simulink model "WiFi"  (Simulink 5.0)
settings: Solver=VariableStepDiscrete  StartTime=0.0  StopTime=inf  RelTol=1e-3
PreLoadFcn:
  | EsNo=18; Distance=.1;
undefined symbols (not defined in the file): CRC_size, Filter_order, Fs, Length_size, Packet_size, PLCP_header_receive_delay, PLCP_header_size, PLCP_preamble_receive_delay, PLCP_preamble_size, PLCP_size, PPDU_frame_period, PPDU_size_chips, PSDU_receive_delay, PSDU_size, randint, Samples_per_chips, Service_size, SFD_size, Signal_size, Sync_bits, Sync_size
libraries: WiFi_lib x8, dspsrcs4 x6, commsink2 x5, dspsigops x4, simulink x3, dspsnks4 x1, dsparch3 x1, commutil2 x1, commrandsrc2 x1, dspmlti3 x1, dspstat3 x1
settings Model: Creator=Stuart Amit  LastModifiedBy=stuartm  SaveTime=off  SaveOutput=off  BooleanDataType=off

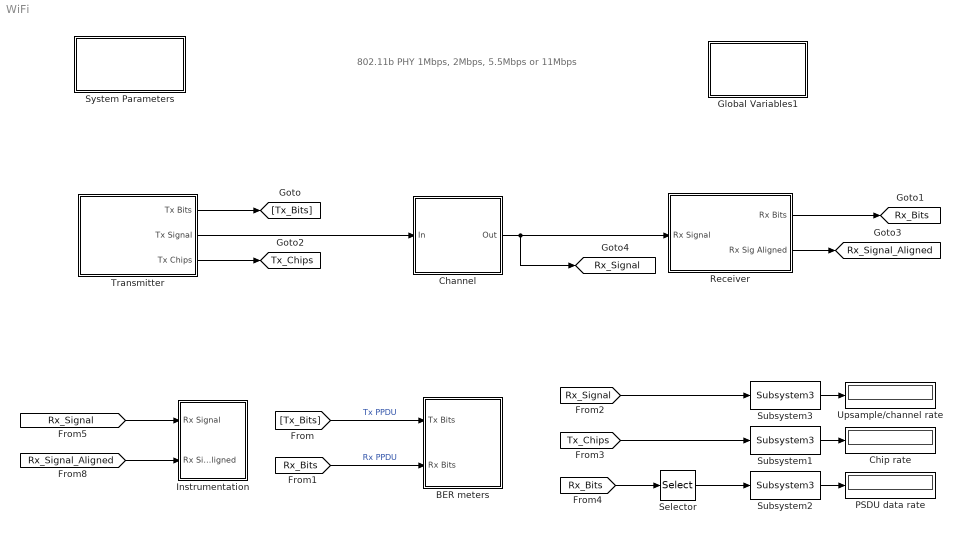
== system WiFi ==
  note: 802.11b PHY
      |   1Mbps, 2Mbps, 5.5Mbps or 11Mbps
  BER meters : Subsystem
  Channel : Subsystem  BlockChoice=AWGN
      settings: AttributesFormatString=%<BlockChoice>  TemplateBlock=WiFi_lib/Channel  MemberBlocks=AWGN,None
  Chip rate : Display
  Global Variables1 : Subsystem
      mask Display: disp('Info')
  Instrumentation : Subsystem  TreatAsAtomicUnit=on  mask(Instrumentation){On=off, Off=on}
      mask init:
      | if strcmp(On,'on')
      |   picture=imread('Switch_On.jpg');
      |   set_param([gcb,'/State'],'Value','1');
      | else
      |   picture=imread('Switch_Off.jpg');
      |   set_param([gcb,'/State'],'Value','0');
      | end
      settings: OpenFcn=temp=get_param(gcb,'On');set_param(gcb,'On', get_param(gcb,'Off'));set_param(gcb,'Off', temp);
      mask Display: image(picture,'center')
  PSDU data rate : Display
  Receiver : Subsystem
  Selector : Selector  Elements=[1: PSDU_size]  InputPortWidth=PPDU_size
  Subsystem1 : WiFi_lib/Subsystem3  Units=MHz
  Subsystem2 : WiFi_lib/Subsystem3  Units=MHz
  Subsystem3 : WiFi_lib/Subsystem3  Units=MHz
  System Parameters : Subsystem  mask(Set System Parameters){Mode=11Mbps, Packet_size=1024, Short_preamble=off, Channel_number=11, Channel_type=AWGN, EsNo=EsNo}
      mask prompts: Mode "Mode/Data Rate"; Packet_size "Packet Size (Bytes)"; Short_preamble "Use Short Preamble"; Channel_number "Channel Number"; Channel_type "Channel Type"; EsNo "Channel EsNo"
      mask help: These system parameters set-up configurable subsystems in the model to implmentedort the requested parameters. Calls wifi_init.m to perfom this task as well as calculate delays.
      mask init:
      | WiFi_init
      settings: AttributesFormatString="Rate = %<Mode>\\nPacket Size = %<Packet_size> Bytes\\nShort Preamble is %<Short_preamble>\\nChannel Number = %<Channel_number>\\nChannel Type =  %<Channel_type>\\nChannel Noise (EsNo) =  %<EsNo> dB\\n"
      mask StyleString: popup(1Mbps|2Mbps|5.5Mbps|11Mbps),edit,checkbox,popup(1|2|3|4|5|6|7|8|9|10|11),popup(None|AWGN),edit
      mask CallbackString:
      | ||||if strcmp(get_param(gcb,'Channel_type'),'AWGN')
      | 	set_param(gcb,'MaskEnables',{'on' 'on' 'on' 'on' 'on' 'on'})
      | else
      | 	set_param(gcb,'MaskEnables',{'on' 'on' 'on' 'on' 'on' 'off'})
      | end
      | 	|
      mask Display: disp('System Parameters')
  Transmitter : Subsystem
  Upsample/channel rate : Display
  tag scope: Rx_Bits=global, Rx_Signal=global, Rx_Signal_Aligned=global, Tx_Chips=global
  wires:
  Transmitter/2(Tx Signal) -> Channel/1(In)
  Transmitter/1(Tx Bits) -> [Tx_Bits]
  Receiver/1(Rx Bits) -> [Rx_Bits]
  [Rx_Bits] -> BER meters/2(Rx Bits)  "Rx PPDU"
  [Tx_Bits] -> BER meters/1(Tx Bits)  "Tx PPDU"
  Channel/1(Out) -> Receiver/1(Rx Signal), [Rx_Signal]
  Subsystem3/1 -> Upsample/channel rate/1
  [Rx_Signal] -> Subsystem3/1
  Subsystem1/1 -> Chip rate/1
  [Tx_Chips] -> Subsystem1/1
  [Rx_Bits] -> Selector/1
  Subsystem2/1 -> PSDU data rate/1
  Selector/1 -> Subsystem2/1
  Receiver/2(Rx Sig Aligned) -> [Rx_Signal_Aligned]
  [Rx_Signal_Aligned] -> Instrumentation/2(Rx Signal Aligned)
  [Rx_Signal] -> Instrumentation/1(Rx Signal)
  Transmitter/3(Tx Chips) -> [Tx_Chips]

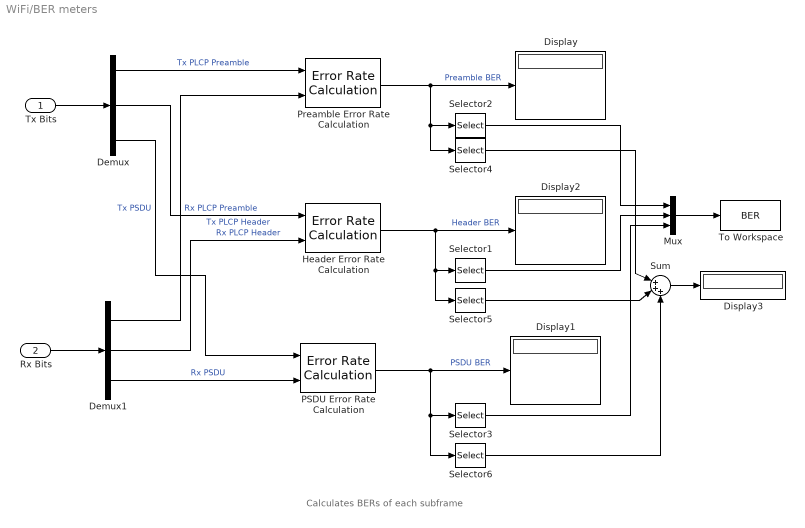
== system WiFi/BER meters ==
  note: Calculates BERs of each subframe
  Tx Bits : Inport
  Rx Bits : Inport  Port=2
  Demux : Demux  Outputs=[PLCP_preamble_size PLCP_header_size PSDU_size]
  Demux1 : Demux  Outputs=[PLCP_preamble_size PLCP_header_size PSDU_size]
  Display{,1..3} (4 alike) : Display
  Header Error Rate Calculation : commsink2/Error Rate Calculation  N=PLCP_header_receive_delay  st_delay=PLCP_header_computation_delay  cp_mode=Entire frame  subframe=3:4808  PMode=Port  WsName=ErrorVec  RsMode2=off  stop=off  numErr=100  maxBits=1e6
  Mux : Mux  Inputs=3
  PSDU Error Rate Calculation : commsink2/Error Rate Calculation  N=PSDU_receive_delay  st_delay=PSDU_computation_delay  cp_mode=Entire frame  subframe=3:4808  PMode=Port  WsName=ErrorVec  RsMode2=off  stop=on  numErr=100  maxBits=1e6
  Preamble Error Rate Calculation : commsink2/Error Rate Calculation  N=PLCP_preamble_receive_delay  st_delay=PLCP_preamble_computation_delay  cp_mode=Entire frame  subframe=3:4808  PMode=Port  WsName=ErrorVec  RsMode2=off  stop=off  numErr=100  maxBits=1e6
  Selector1 : Selector  Elements=[1]  InputPortWidth=3
  Selector2 : Selector  Elements=[1]  InputPortWidth=3
  Selector3 : Selector  Elements=[1]  InputPortWidth=3
  Selector4 : Selector  Elements=3  InputPortWidth=3
  Selector5 : Selector  Elements=3  InputPortWidth=3
  Selector6 : Selector  Elements=3  InputPortWidth=3
  Sum : Sum  Inputs=|+++  SaturateOnIntegerOverflow=on  InputSameDT=on
  To Workspace : ToWorkspace  VariableName=BER  SampleTime=-1  SaveFormat=Array
      settings: MaxDataPoints=1
  wires:
  Preamble Error Rate Calculation/1 -> Display/1, Selector2/1, Selector4/1  "Preamble BER"
  PSDU Error Rate Calculation/1 -> Display1/1, Selector3/1, Selector6/1  "PSDU BER"
  Demux1/1 -> Preamble Error Rate Calculation/2  "Rx PLCP Preamble"
  Demux/1 -> Preamble Error Rate Calculation/1  "Tx PLCP Preamble"
  Header Error Rate Calculation/1 -> Display2/1, Selector1/1, Selector5/1  "Header BER"
  Demux1/3 -> PSDU Error Rate Calculation/2  "Rx PSDU"
  Demux/3 -> PSDU Error Rate Calculation/1  "Tx PSDU"
  Demux/2 -> Header Error Rate Calculation/1  "Tx PLCP Header"
  Demux1/2 -> Header Error Rate Calculation/2  "Rx PLCP Header"
  Tx Bits/1 -> Demux/1
  Rx Bits/1 -> Demux1/1
  Selector2/1 -> Mux/1
  Mux/1 -> To Workspace/1
  Selector1/1 -> Mux/2
  Selector3/1 -> Mux/3
  Sum/1 -> Display3/1
  Selector4/1 -> Sum/1
  Selector5/1 -> Sum/2
  Selector6/1 -> Sum/3

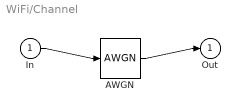
== system WiFi/Channel ==
  In : Inport
  AWGN : WiFi_lib/AWGN
  Out : Outport
  wires:
  In/1 -> AWGN/1
  AWGN/1 -> Out/1

== system WiFi/Global Variables1 ==
  note: Implements: IEEE Std 802.11b-1999 PHY
      | (Supplement to ANSI/IEEE Std 802.11, 1999 Edition)
      | Available from: http://standards.ieee.org/reading/ieee/std/lanman/
      |
      | System Parameters: Double click block to display and set
      |
      | * Mode/Data Rate: Choose from 1Mpbs, 2Mbps, 5.5Mbps or 11Mbps
      | * Packet size: 1-4095 Bytes
      | * Use short preamble: An option for 2, 5.5 or 11Mbps options only
      | * Channel number: Select from 1 to 11
      | * Channel type: None or AWGN
      | * EsNo: Channel noise power for AWGN option

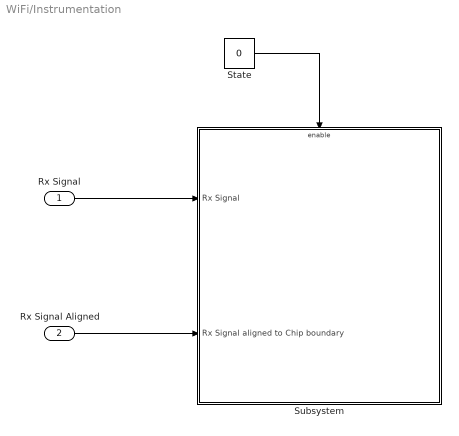
== system WiFi/Instrumentation ==
  Rx Signal : Inport
  Rx Signal Aligned : Inport  Port=2
  State : Constant  Value=0
  Subsystem : Subsystem  TreatAsAtomicUnit=on
  wires:
  State/1 -> Subsystem/Enable
  Rx Signal Aligned/1 -> Subsystem/2(Rx Signal aligned to Chip boundary)
  Rx Signal/1 -> Subsystem/1("Rx Signal ")

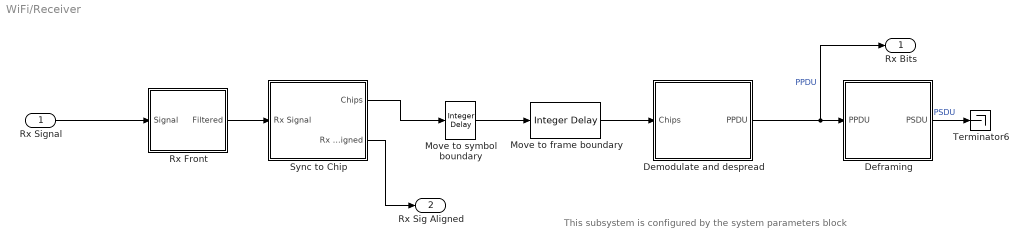
== system WiFi/Receiver ==
  note: This subsystem is configured
      | by the system parameters block
  Rx Signal : Inport
  Deframing : Subsystem
  Demodulate and despread : Subsystem  BlockChoice=11Mbps demod
      link override 11Mbps demod: Short_preamble=off
      link override 11Mbps demod/PLCP demod: BlockChoice=PLCP demod for long preamble
      link override 1Mbps demod/PLCP demod: BlockChoice=PLCP demod for short preamble
      link override 2Mbps demod: Short_preamble=off
      link override 2Mbps demod/PLCP demod: BlockChoice=PLCP demod for long preamble
      link override 5.5Mbps demod: Short_preamble=off
      link override 5.5Mbps demod/PLCP demod: BlockChoice=PLCP demod for long preamble
      settings: AttributesFormatString=%<BlockChoice>  TemplateBlock=WiFi_lib/Demodulate and despread  MemberBlocks=11Mbps demod,1Mbps demod,2Mbps demod,5.5Mbps demod
  "Move to frame boundary " : dspsigops/Integer Delay  delay=PPDU_size_chips-11  ic=0  reset_popup=None
  "Move to symbol boundary " : dspsigops/Integer Delay  delay=Filter_delay_chips_correction  ic=0  reset_popup=None
  Rx Front : Subsystem
  Sync to Chip : Subsystem
  Terminator6 : Terminator
  Rx Bits : Outport
  Rx Sig Aligned : Outport  Port=2
  wires:
  Sync to Chip/1(Chips) -> "Move to symbol boundary "/1
  "Move to symbol boundary "/1 -> "Move to frame boundary "/1
  "Move to frame boundary "/1 -> Demodulate and despread/1(Chips)
  Rx Signal/1 -> Rx Front/1(Signal)
  Deframing/1(PSDU) -> Terminator6/1  "PSDU"
  Demodulate and despread/1(PPDU) -> Deframing/1(PPDU), Rx Bits/1  "PPDU"
  Rx Front/1(Filtered) -> Sync to Chip/1(Rx Signal)
  Sync to Chip/2(Rx Signal Aligned) -> Rx Sig Aligned/1

== system WiFi/System Parameters ==

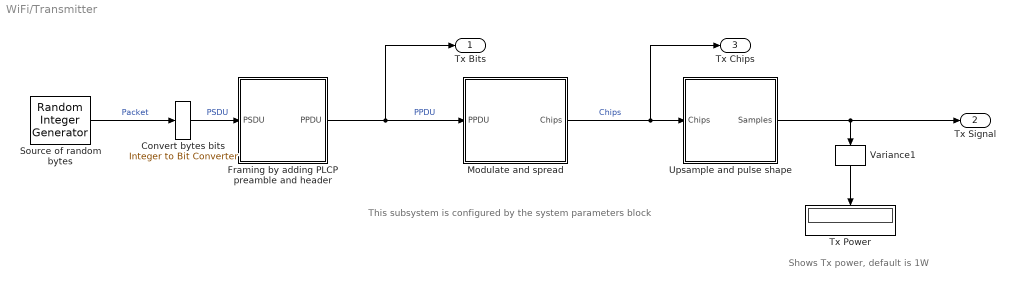
== system WiFi/Transmitter ==
  note: This subsystem is configured
      | by the system parameters block
  note: Shows Tx power, default is 1W
  Convert bytes bits : commutil2/Integer to Bit Converter  nbits=8
  Framing by adding PLCP preamble and header : Subsystem
  Modulate and spread : Subsystem  BlockChoice=11Mbps mod
      link override 11Mbps mod: Short_preamble=off
      link override 11Mbps mod/PLCP mod: BlockChoice=PLCP mod for long preamble
      link override 1Mbps mod/PLCP mod: BlockChoice=PLCP mod for short preamble
      link override 2Mbps mod: Short_preamble=off
      link override 2Mbps mod/PLCP mod: BlockChoice=PLCP mod for long preamble
      link override 5.5Mbps mod: Short_preamble=off
      link override 5.5Mbps mod/PLCP mod: BlockChoice=PLCP mod for long preamble
      settings: AttributesFormatString=%<BlockChoice>  TemplateBlock=WiFi_lib/Modulate and spread  MemberBlocks=11Mbps mod,1Mbps mod,2Mbps mod,5.5Mbps mod
  Source of random bytes : commrandsrc2/Random Integer Generator  mul=255  seed=[12345]  Ts=PPDU_frame_period/Packet_size  frameBased=on  sampPerFrame=Packet_size  orient=off
  Tx Power : Display
      settings: Orientation=down
  Upsample and pulse shape : Subsystem
  Variance1 : dspstat3/Variance  Orientation=down  run=off  reset_popup=None
  Tx Bits : Outport
  Tx Signal : Outport  Port=2
  Tx Chips : Outport  Port=3
  wires:
  Source of random bytes/1 -> Convert bytes bits/1  "Packet"
  Convert bytes bits/1 -> Framing by adding PLCP preamble and header/1(PSDU)  "PSDU"
  Framing by adding PLCP preamble and header/1(PPDU) -> Tx Bits/1, Modulate and spread/1(PPDU)  "PPDU"
  Upsample and pulse shape/1(Samples) -> Variance1/1, Tx Signal/1
  Modulate and spread/1(Chips) -> Upsample and pulse shape/1(Chips), Tx Chips/1  "Chips"
  Variance1/1 -> Tx Power/1

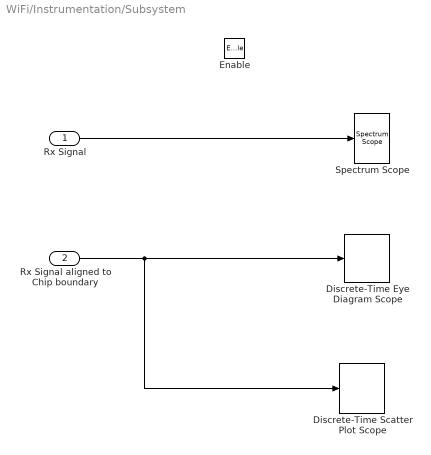
== system WiFi/Instrumentation/Subsystem ==
  "Rx Signal " : Inport
  Rx Signal aligned to Chip boundary : Inport  Port=2
  Enable : EnablePort
  Discrete-Time Eye Diagram Scope : commsink2/Discrete-Time Eye Diagram Scope  Tag=EyeDiagram  showPlotting=off  sampPerSymb=8  offsetEye=0  symbPerTrace=1  numTraces=40  numNewFrames=40  showRendering=off  LineStyles=-  LineColors=b  dupPoints=on  fading=on  render=on  AxisGrid=off  showAxes=off  yMin=-1.38526904502056  yMax=1.38777979583567  inphaseLabel=In-phase Amplitude  quadratureLabel=Quadrature Amplitude  showFigure=on  openScopeAtSimStart=on  dispDiagram=In-phase and Quadrature  FrameNumber=off  FigPos=[22 40 434 377]  figTitle=Rx Signal  block_type_=eye  numLinesMax=8
  Discrete-Time Scatter Plot Scope : commsink2/Discrete-Time Scatter Plot Scope  Tag=ScatterPlot  showPlotting=on  sampPerSymb=8  offsetEye=0  numTraces=100  numNewFrames=100  showRendering=off  LineMarkers=.  LineColors=b  fading=on  render=on  AxisGrid=on  showAxes=off  xMin=-1  xMax=1  yMin=-1  yMax=1  inphaseLabel=In-phase Amplitude  quadratureLabel=Quadrature Amplitude  showFigure=off  openScopeAtSimStart=on  FrameNumber=off  FigPos=[556 40 356 359]  figTitle=Rx Chips  numLinesMax=8  block_type_=scatter
  Spectrum Scope : dspsnks4/Spectrum Scope  ScopeProperties=on  Domain=Frequency  HorizSpan=1  UseBuffer=on  BufferSize=1024  Overlap=0  inpFftLenInherit=on  FFTlength=1024  numAvg=5  DisplayProperties=off  AxisGrid=on  Memory=off  FrameNumber=on  AxisLegend=off  AxisZoom=off  OpenScopeAtSimStart=on  OpenScopeImmediately=off  FigPos=[23 469 431 222]  AxisProperties=off  XUnits=Hertz  XRange=[-Fs/2...Fs/2]  InheritXIncr=on  XIncr=1.0  XLabel=Samples  YUnits=dB  YLabel=Magnitude, dB  LineProperties=off  LineStyles=--
      settings: YMin=-20.2099642477694  YMax=13.0534015069536
  wires:
  Rx Signal aligned to Chip boundary/1 -> Discrete-Time Scatter Plot Scope/1, Discrete-Time Eye Diagram Scope/1
  "Rx Signal "/1 -> Spectrum Scope/1

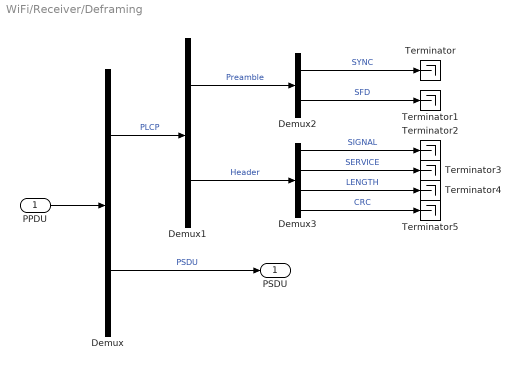
== system WiFi/Receiver/Deframing ==
  PPDU : Inport
  Demux : Demux  Outputs=[PLCP_size PSDU_size]
  Demux1 : Demux  Outputs=[PLCP_preamble_size PLCP_header_size]
  Demux2 : Demux  Outputs=[Sync_size SFD_size]
  Demux3 : Demux  Outputs=[Signal_size Service_size Length_size CRC_size]
  Terminator{,1..5} (6 alike) : Terminator
  PSDU : Outport
  wires:
  Demux2/1 -> Terminator/1  "SYNC"
  Demux2/2 -> Terminator1/1  "SFD"
  Demux3/1 -> Terminator2/1  "SIGNAL"
  Demux3/2 -> Terminator3/1  "SERVICE"
  Demux3/3 -> Terminator4/1  "LENGTH"
  Demux3/4 -> Terminator5/1  "CRC"
  PPDU/1 -> Demux/1
  Demux1/2 -> Demux3/1  "Header"
  Demux1/1 -> Demux2/1  "Preamble"
  Demux/1 -> Demux1/1  "PLCP"
  Demux/2 -> PSDU/1  "PSDU"

== system WiFi/Receiver/Demodulate and despread ==
  Chips : Inport
  11Mbps demod : WiFi_lib/11Mbps demod  Short_preamble=off
  PPDU : Outport
  wires:
  Chips/1 -> 11Mbps demod/1
  11Mbps demod/1 -> PPDU/1

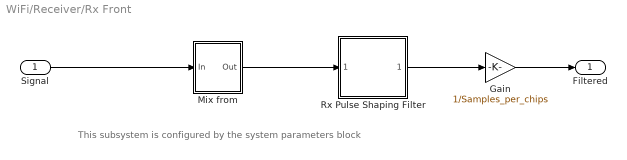
== system WiFi/Receiver/Rx Front ==
  note: This subsystem is configured
      | by the system parameters block
  Signal : Inport
  Gain : Gain  Gain=1/Samples_per_chips  SaturateOnIntegerOverflow=on
  Mix from : Subsystem  BlockChoice=Mix from center frequency
      link override Mix from center frequency/Vector Scope: OpenScopeImmediately=off  LineColors=[1 0 0]  LineStyles=--|--  FigPos=[75 73 830 420]
      settings: AttributesFormatString=%<BlockChoice>  TemplateBlock=WiFi_lib/Mix from  MemberBlocks=Mix from center frequency,No mix from center frequency
      link override Mix from center frequency/Vector Scope: YMin=-1.35082863252636  YMax=1.35082863252639
  Rx Pulse Shaping Filter : Subsystem  mask(Tx FIR Pulse Shaping Filter){numTaps=Filter_order, beta=.3, N=Samples_per_chips}
      mask prompts: numTaps "Number of Filter Taps:"; beta "RRC Roll-off Factor:"; N "Oversampling Factor:"
      mask help: The pulse shaping filter consits of a RRC (Root Raised Cosinus) with roll-off factor of 0.22. The length of the FIR filter is 96 coeffcients.
      mask init:
      | h=N*firrcos(numTaps,5e6,beta,88e6,'rolloff','sqrt',numTaps/2,kaiser(numTaps+1,1));
      | assignin('base','h',h );
      mask Display: plot( 1:prod( size( h)), h);
  Filtered : Outport
  wires:
  Signal/1 -> Mix from/1(In)
  Mix from/1(Out) -> Rx Pulse Shaping Filter/1("   ")
  Rx Pulse Shaping Filter/1(" ") -> Gain/1
  Gain/1 -> Filtered/1

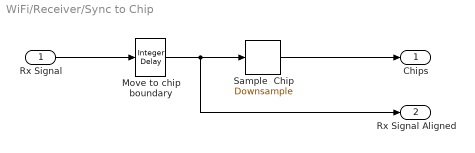
== system WiFi/Receiver/Sync to Chip ==
  Rx Signal : Inport
  Move to chip boundary : dspsigops/Integer Delay  delay=Filter_delay_samples_correction  ic=0  reset_popup=None
  Sample  Chip : dspsigops/Downsample  N=Samples_per_chips  phase=0  ic=0  smode=Allow multirate  fmode=Maintain input frame size
  Chips : Outport
  Rx Signal Aligned : Outport  Port=2
  wires:
  Move to chip boundary/1 -> Sample  Chip/1, Rx Signal Aligned/1
  Sample  Chip/1 -> Chips/1
  Rx Signal/1 -> Move to chip boundary/1

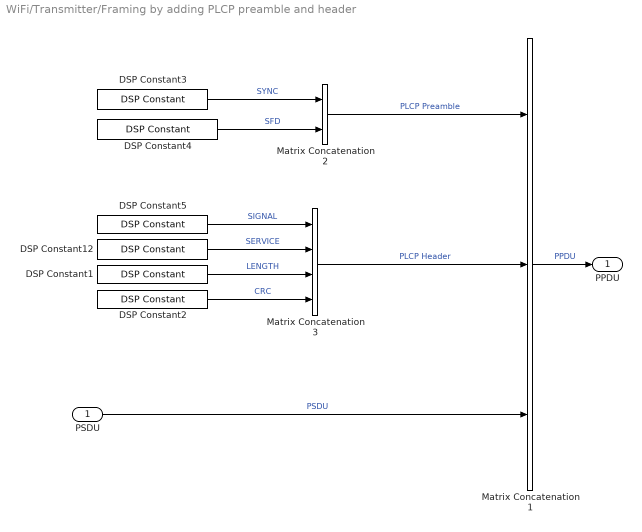
== system WiFi/Transmitter/Framing by adding PLCP preamble and header ==
  PSDU : Inport
  DSP Constant1 : dspsrcs4/DSP Constant  Value=randint(Length_size,1)  SampleMode=Discrete  discreteOutput=Frame-based  continuousOutput=Sample-based  sampTime=PPDU_frame_period  framePeriod=PPDU_frame_period  dataType=Inherit from 'Constant value'  wordLen=16  udDataType=sfix(16)  fracBitsMode=Best precision  numFracBits=15  InterpretAs1D=off  Ts=PPDU_frame_period  FramebasedOutput=on
  DSP Constant12 : dspsrcs4/DSP Constant  Value=zeros(Service_size,1)  SampleMode=Discrete  discreteOutput=Frame-based  continuousOutput=Sample-based  sampTime=PPDU_frame_period  framePeriod=PPDU_frame_period  dataType=Inherit from 'Constant value'  wordLen=16  udDataType=sfix(16)  fracBitsMode=Best precision  numFracBits=15  InterpretAs1D=off  Ts=PPDU_frame_period  FramebasedOutput=on
  DSP Constant2 : dspsrcs4/DSP Constant  Value=randint(CRC_size,1)  SampleMode=Discrete  discreteOutput=Frame-based  continuousOutput=Sample-based  sampTime=PPDU_frame_period  framePeriod=PPDU_frame_period  dataType=Inherit from 'Constant value'  wordLen=16  udDataType=sfix(16)  fracBitsMode=Best precision  numFracBits=15  InterpretAs1D=off  Ts=PPDU_frame_period  FramebasedOutput=on
  DSP Constant3 : dspsrcs4/DSP Constant  Value=Sync_bits %ones(Sync_size,1)  SampleMode=Discrete  discreteOutput=Frame-based  continuousOutput=Sample-based  sampTime=PPDU_frame_period  framePeriod=PPDU_frame_period  dataType=Inherit from 'Constant value'  wordLen=16  udDataType=sfix(16)  fracBitsMode=Best precision  numFracBits=15  InterpretAs1D=off  Ts=PPDU_frame_period  FramebasedOutput=on
  DSP Constant4 : dspsrcs4/DSP Constant  Value=de2bi(hex2dec('F3A0'))'  SampleMode=Discrete  discreteOutput=Frame-based  continuousOutput=Sample-based  sampTime=PPDU_frame_period  framePeriod=PPDU_frame_period  dataType=Inherit from 'Constant value'  wordLen=16  udDataType=sfix(16)  fracBitsMode=Best precision  numFracBits=15  InterpretAs1D=off  Ts=PPDU_frame_period  FramebasedOutput=on
  DSP Constant5 : dspsrcs4/DSP Constant  Value=zeros(Signal_size,1)  SampleMode=Discrete  discreteOutput=Frame-based  continuousOutput=Sample-based  sampTime=PPDU_frame_period  framePeriod=PPDU_frame_period  dataType=Inherit from 'Constant value'  wordLen=16  udDataType=sfix(16)  fracBitsMode=Best precision  numFracBits=15  InterpretAs1D=off  Ts=PPDU_frame_period  FramebasedOutput=on
  Matrix Concatenation1 : simulink/Math Operations/Matrix Concatenation  numInports=3  catMethod=Vertical
  Matrix Concatenation2 : simulink/Math Operations/Matrix Concatenation  numInports=2  catMethod=Vertical
  Matrix Concatenation3 : simulink/Math Operations/Matrix Concatenation  numInports=4  catMethod=Vertical
  PPDU : Outport
  wires:
  DSP Constant3/1 -> Matrix Concatenation2/1  "SYNC"
  DSP Constant4/1 -> Matrix Concatenation2/2  "SFD"
  DSP Constant5/1 -> Matrix Concatenation3/1  "SIGNAL"
  DSP Constant12/1 -> Matrix Concatenation3/2  "SERVICE"
  DSP Constant1/1 -> Matrix Concatenation3/3  "LENGTH"
  DSP Constant2/1 -> Matrix Concatenation3/4  "CRC"
  Matrix Concatenation3/1 -> Matrix Concatenation1/2  "PLCP Header"
  Matrix Concatenation1/1 -> PPDU/1  "PPDU"
  PSDU/1 -> Matrix Concatenation1/3  "PSDU"
  Matrix Concatenation2/1 -> Matrix Concatenation1/1  "PLCP Preamble"

== system WiFi/Transmitter/Modulate and spread ==
  PPDU : Inport
  11Mbps mod : WiFi_lib/11Mbps mod  Short_preamble=off
  Chips : Outport
  wires:
  PPDU/1 -> 11Mbps mod/1
  11Mbps mod/1 -> Chips/1

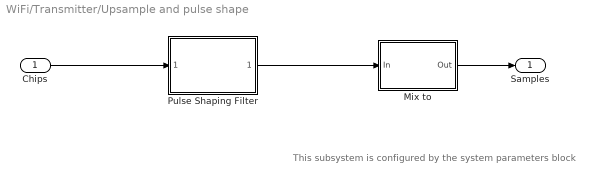
== system WiFi/Transmitter/Upsample and pulse shape ==
  note: This subsystem is configured
      | by the system parameters block
  Chips : Inport
  Mix to : Subsystem  BlockChoice=Mix to center frequency
      settings: AttributesFormatString=%<BlockChoice>  TemplateBlock=WiFi_lib/Mix to  MemberBlocks=Mix to center frequency,No mix to center frequency
  Pulse Shaping Filter : Subsystem  mask(Tx FIR Pulse Shaping Filter){numTaps=Filter_order, beta=.3, N=Samples_per_chips}
      mask prompts: numTaps "Number of Filter Taps:"; beta "RRC Roll-off Factor:"; N "Oversampling Factor:"
      mask help: The pulse shaping filter consits of a RRC (Root Raised Cosinus) with roll-off factor of 0.22. The length of the FIR filter is 96 coeffcients.
      mask init:
      | h=N*firrcos(numTaps,5e6,beta,88e6,'rolloff','sqrt',numTaps/2,kaiser(numTaps+1,1));
      | assignin('base','h',h );
      mask Display: plot( 1:prod( size( h)), h);
  Samples : Outport
  wires:
  Chips/1 -> Pulse Shaping Filter/1("   ")
  Mix to/1(Out) -> Samples/1
  Pulse Shaping Filter/1(" ") -> Mix to/1(In)

== system WiFi/Receiver/Rx Front/Mix from ==
  In : Inport
  Mix from center frequency : WiFi_lib/Mix from center frequency  SimViewingDevice=off  DataTypeOverride=UseLocalSettings  MinMaxOverflowLogging=UseLocalSettings
      settings: Permissions=ReadWrite  RTWFcnNameOpts=Auto  RTWFileNameOpts=Auto
  Out : Outport
  wires:
  In/1 -> Mix from center frequency/1
  Mix from center frequency/1 -> Out/1

== system WiFi/Receiver/Rx Front/Rx Pulse Shaping Filter ==
  "   " : Inport
  Direct-Form II Transpose Filter : dsparch3/Direct-Form II Transpose Filter  num=h  den=1  ic=0
  " " : Outport
  wires:
  "   "/1 -> Direct-Form II Transpose Filter/1
  Direct-Form II Transpose Filter/1 -> " "/1

== system WiFi/Transmitter/Upsample and pulse shape/Mix to ==
  In : Inport
  Mix to center frequency : WiFi_lib/Mix to center frequency  SimViewingDevice=off  DataTypeOverride=UseLocalSettings  MinMaxOverflowLogging=UseLocalSettings
      settings: Permissions=ReadWrite  RTWFcnNameOpts=Auto  RTWFileNameOpts=Auto
  Out : Outport
  wires:
  In/1 -> Mix to center frequency/1
  Mix to center frequency/1 -> Out/1

== system WiFi/Transmitter/Upsample and pulse shape/Pulse Shaping Filter ==
  "   " : Inport
  FIR Interpolation : dspmlti3/FIR Interpolation  h=h  L=N  framing=Maintain input frame size  outputBufInitCond=0
  " " : Outport
  wires:
  FIR Interpolation/1 -> " "/1
  "   "/1 -> FIR Interpolation/1
